simulink model "UDE"  (R2020a)
settings: Solver=ode4  StartTime=0.0  StopTime=tstop  FixedStep=tstep  RelTol=1e-3
values from neighbouring files (symbols this model uses):
  tracking_ic = (1/p)*(refT - q*x_hat_ic)    [data.m]
  Ts = 0.01    [data.m]
  ua_ic = -Ad(2, :)*TC*x_hat_ic    [data.m]
  x_hat_ic = [-2; 1]    [data.m]
  xic = [-3 2]'    [data.m]
settings Model: Creator=Ram Padmanabhan  LastModifiedBy=Ram Padmanabhan
settings DataIOCC: SaveOutput=off  SignalLogging=off  DSMLogging=off  SaveTime=off  ReturnWorkspaceOutputs=off

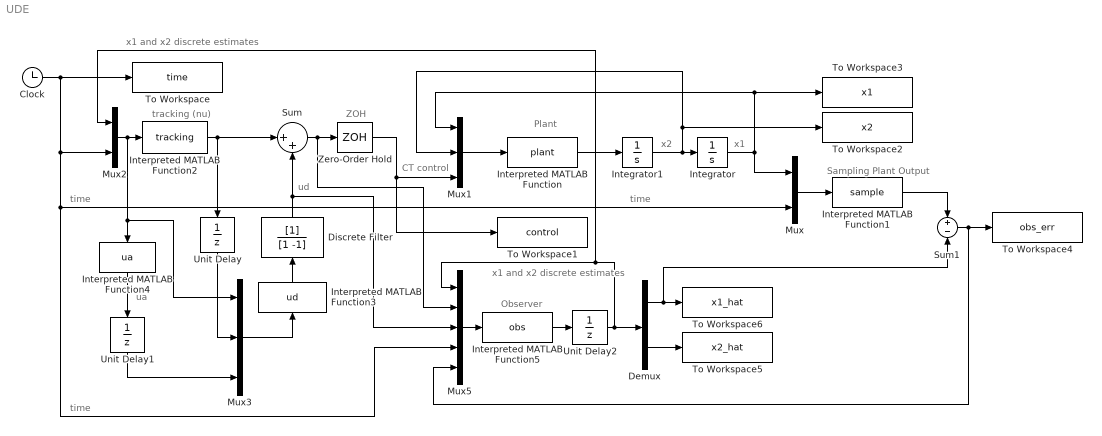
== system UDE ==
  note: time
  note: Plant
  note: CT control
  note: ZOH
  note: ud
  note: ua
  note: tracking (nu)
  note: Sampling Plant Output
  note: x1
  note: x2
  note: Observer
  note: x1 and x2 discrete estimates
  note: time
  note: time
  note: x1 and x2 discrete estimates
  Clock : Clock
  Demux : Demux  Outputs=2
  Discrete Filter : DiscreteFilter  Denominator=[1 -1]  SampleTime=Ts
  Integrator : Integrator  InitialCondition=xic(1)
  Integrator1 : Integrator  InitialCondition=xic(2)
  Interpreted MATLAB Function : MATLABFcn  MATLABFcn=plant  OutputDimensions=1
  Interpreted MATLAB Function1 : MATLABFcn  MATLABFcn=sample  OutputDimensions=1
  Interpreted MATLAB Function2 : MATLABFcn  MATLABFcn=tracking  OutputDimensions=1
  Interpreted MATLAB Function3 : MATLABFcn  MATLABFcn=ud  OutputDimensions=1
  Interpreted MATLAB Function4 : MATLABFcn  MATLABFcn=ua  OutputDimensions=1
  Interpreted MATLAB Function5 : MATLABFcn  MATLABFcn=obs  OutputDimensions=2  Output1D=off
  Mux : Mux  Inputs=2
  Mux1 : Mux  Inputs=3
  Mux2 : Mux  Inputs=2
  Mux3 : Mux  Inputs=3
  Mux5 : Mux  Inputs=5
  Sum : Sum  Inputs=|++
  Sum1 : Sum  Inputs=+-
  To Workspace : ToWorkspace  VariableName=time  SampleTime=-1
  To Workspace1 : ToWorkspace  VariableName=control  SampleTime=-1
  To Workspace2 : ToWorkspace  VariableName=x2  SampleTime=-1
  To Workspace3 : ToWorkspace  VariableName=x1  SampleTime=-1
  To Workspace4 : ToWorkspace  VariableName=obs_err  SampleTime=-1
  To Workspace5 : ToWorkspace  VariableName=x2_hat  SampleTime=-1
  To Workspace6 : ToWorkspace  VariableName=x1_hat  SampleTime=-1
  Unit Delay : UnitDelay  InitialCondition=tracking_ic  SampleTime=Ts  HasFrameUpgradeWarning=on
  Unit Delay1 : UnitDelay  InitialCondition=ua_ic  SampleTime=Ts  HasFrameUpgradeWarning=on
  Unit Delay2 : UnitDelay  InitialCondition=x_hat_ic  SampleTime=Ts  HasFrameUpgradeWarning=on
  Zero-Order Hold : ZeroOrderHold  SampleTime=Ts
  wires:
  Integrator1/1 -> To Workspace2/1, Mux1/2, Integrator/1
  Interpreted MATLAB Function/1 -> Integrator1/1
  Integrator/1 -> Mux/1, Mux1/1, To Workspace3/1
  Mux/1 -> Interpreted MATLAB Function1/1
  Clock/1 -> Mux5/4, Mux/2, Mux2/2, To Workspace/1
  Mux1/1 -> Interpreted MATLAB Function/1
  Interpreted MATLAB Function2/1 -> Sum/1, Unit Delay/1
  Interpreted MATLAB Function3/1 -> Discrete Filter/1
  Zero-Order Hold/1 -> Mux1/3, To Workspace1/1
  Sum/1 -> Mux5/2, Zero-Order Hold/1
  Demux/2 -> To Workspace5/1
  Demux/1 -> To Workspace6/1, Sum1/2
  Mux5/1 -> Interpreted MATLAB Function5/1
  Sum1/1 -> To Workspace4/1, Mux5/5
  Discrete Filter/1 -> Mux5/3, Sum/2
  Interpreted MATLAB Function4/1 -> Unit Delay1/1
  Mux2/1 -> Interpreted MATLAB Function2/1, Interpreted MATLAB Function4/1, Mux3/1
  Mux3/1 -> Interpreted MATLAB Function3/1
  Interpreted MATLAB Function1/1 -> Sum1/1
  Interpreted MATLAB Function5/1 -> Unit Delay2/1
  Unit Delay2/1 -> Demux/1, Mux2/1, Mux5/1
  Unit Delay1/1 -> Mux3/3
  Unit Delay/1 -> Mux3/2
